simulink model "Nonlinear_UIO"  (R2020b)
settings: Solver=ode4  StartTime=0.0  StopTime=20  FixedStep=0.0001  RelTol=1e-3
values from neighbouring files (symbols this model uses):
  E = U + Y*V    [NUIO_Paper_Implementation_Script.m]
  L = K*(eye(size(C*E)) + C*E) - M*A*E    [NUIO_Paper_Implementation_Script.m]
  M = eye(size(E*C)) + E*C    [NUIO_Paper_Implementation_Script.m]
  N = M*A - K*C    [NUIO_Paper_Implementation_Script.m]
  z_intial = [3;3;3]    [NUIO_Paper_Implementation_Script.m]
settings Model: Creator=sanjay  LastModifiedBy=Sanjay
settings DebuggingCC: AlgebraicLoopMsg=none

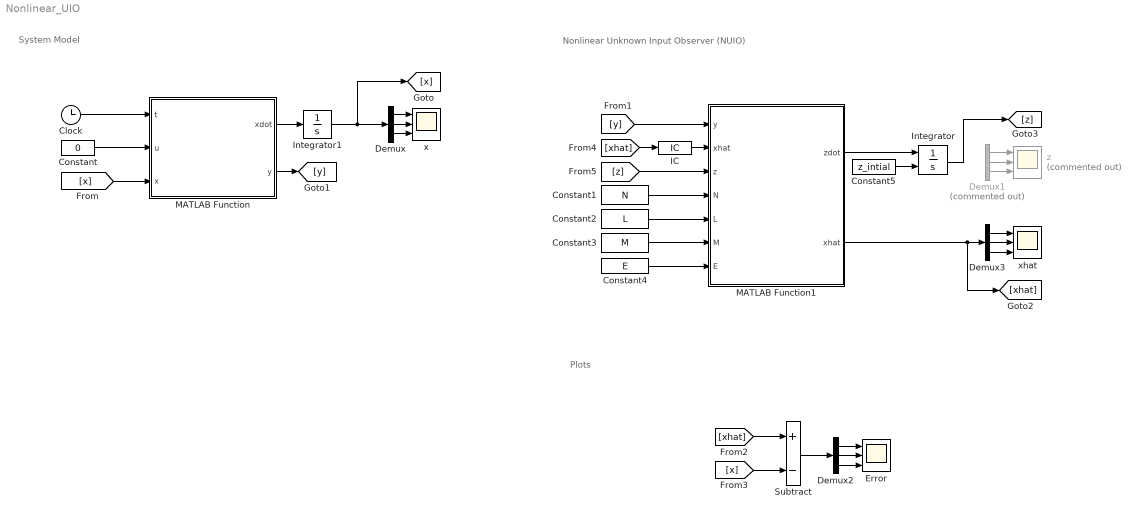
== system Nonlinear_UIO ==
  note: Plots
  note: Nonlinear Unknown Input Observer (NUIO)
  note: System Model
  Clock : Clock
  Constant : Constant  Value=0
  Constant1 : Constant  Value=N
  Constant2 : Constant  Value=L
  Constant3 : Constant  Value=M
  Constant4 : Constant  Value=E
  Constant5 : Constant  Value=z_intial
  Demux : Demux  Outputs=3
  Demux1 : Demux  Commented=on  Outputs=3
  Demux2 : Demux  Outputs=3
  Demux3 : Demux  Outputs=3
  Error : Scope  NumInputPorts=3
  IC : InitialCondition  Value=[0;0;0]
  Integrator : Integrator  InitialConditionSource=external  InitialCondition=[3;3;3]
  Integrator1 : Integrator  InitialCondition=[0;0;0]
  MATLAB Function : MATLAB Function  TreatAsAtomicUnit=on
  MATLAB Function1 : MATLAB Function  TreatAsAtomicUnit=on
  Subtract : Sum  Inputs=+-
  x : Scope  NumInputPorts=3
  xhat : Scope  NumInputPorts=3
  z : Scope  Commented=on  NumInputPorts=3
  wires:
  MATLAB Function/2(y) -> [y]
  MATLAB Function1/1(zdot) -> Integrator/1
  MATLAB Function/1(xdot) -> Integrator1/1
  Clock/1 -> MATLAB Function/1(t)
  Constant/1 -> MATLAB Function/2(u)
  Integrator1/1 -> Demux/1, [x]
  [xhat] -> IC/1
  Constant1/1 -> MATLAB Function1/4(N)
  Constant2/1 -> MATLAB Function1/5(L)
  Constant3/1 -> MATLAB Function1/6(M)
  Constant4/1 -> MATLAB Function1/7(E)
  Demux/2 -> x/2
  Demux/1 -> x/1
  Demux/3 -> x/3
  Demux1/3 -> z/3
  Demux1/1 -> z/1
  Demux1/2 -> z/2
  Integrator/1 -> [z]
  Demux2/2 -> Error/2
  Demux2/1 -> Error/1
  Demux2/3 -> Error/3
  Demux3/2 -> xhat/2
  Demux3/1 -> xhat/1
  Demux3/3 -> xhat/3
  Subtract/1 -> Demux2/1
  Constant5/1 -> Integrator/2
  [x] -> MATLAB Function/3(x)
  [y] -> MATLAB Function1/1(y)
  [xhat] -> Subtract/1
  [x] -> Subtract/2
  [z] -> MATLAB Function1/3(z)
  MATLAB Function1/2(xhat) -> [xhat], Demux3/1
  IC/1 -> MATLAB Function1/2("xhat ")

== matlab function Nonlinear_UIO/MATLAB Function1 ==
  data: y input; zdot output; xhat output; xhat input; z input; N input; L input; M input; E input
function [zdot,xhat] = NUIO(y,xhat,z,N,L,M,E)

%%
x2hat = xhat(2); x3hat = xhat(3);

fxhat = [0.5*sin(x2hat); 0.6*cos(x3hat); 0];

zdot = N*z + L*y + M*fxhat;
xhat = z - E*y;

== matlab function Nonlinear_UIO/MATLAB Function ==
  data: t input; xdot output; u input; y output; x input
function [xdot, y] = System(t,u,x)

%% system matrices
A = [-1 -1 0;-1 0 0;0 -1 -1];
B = [0;0;0];
C = [1 0 0;0 0 1];
D = [-1;0;0];

x2 = x(2); x3 = x(3);

fx = [0.5*sin(x2); 0.6*cos(x3); 0];
v = 2*sin(5*t);

%% dynamics
xdot = A*x + B*u + fx + D*v;
y = C*x;
